simulink model "trackVehicleNewVer7_SonarPath"  (R2017b)
settings: Solver=ode45  StartTime=0.0  StopTime=200  FixedStep=0.1  RelTol=1e-3  EnableMultiTasking=on
PreLoadFcn:
  | RTWConfigurationCB('preloadfcn', bdroot);
InitFcn:
  | parameterVehicle
  | parameterObstacles
  | parameterGNC
  | parameterOccupancyGrid
  | parameterPathPlanner
  | parameterWaypointGenerator
  | miscParameters
StopFcn:
  | myAnimationSonarPath(xActEst,yActEst,thetaActEst,X_array, Y_array, rp1,rp2,sonarInfo, obstaclesArray, OccGrid, gridorig, cellsize)
values from neighbouring files (symbols this model uses):
  b = (92/70)*.31    (= 0.407428571429)    [parameterVehicle.m]
  bDR = b    [parameterGNC.m]
  dcArray = [-100 -11 -10 0 10 11 100]    [parameterVehicle.m]
  dcArrayDR = [-100 -11 -10 0 10 11 100]    [parameterGNC.m]
  eTick = 237    [parameterVehicle.m]
  eTickDR = eTick    [parameterGNC.m]
  KP1 = 10    [parameterGNC.m]
  KP2 = 3    [parameterGNC.m]
  maxgoaldist = 0.2    [parameterWaypointGenerator.m]
  maxwaydist = 0.5    [parameterWaypointGenerator.m]
  obstaclesArray = [0; 0; 0]    [miscParameters.m]
  rl = 0.99*rNominal    (= 0.05242941)    [parameterVehicle.m]
  rNominalDR = rNominal    [parameterGNC.m]
  rp1 = 0.3    [parameterGNC.m]
  rr = 1*rNominal    (= 0.052959)    [parameterVehicle.m]
  Tau1 = 0.01    [parameterGNC.m]
  Tau2 = 0.1    [parameterGNC.m]
  TauEncoderDR = 0.1    [parameterGNC.m]
  thetaIC = 0*(pi/180)    (= 0)    [parameterVehicle.m]
  Tsample = 1/10    (= 0.1)    [parameterGNC.m]
  TsampleEncoder = 1/10    (= 0.1)    [parameterVehicle.m]
  TsampleEncoderDR = TsampleEncoder    [parameterGNC.m]
  Vcom = 3*VmaxDR/4    (= 0.361125)    [parameterGNC.m]
  wArray = [-Vmax, -Vmin, 0, 0,   0, Vmin, Vmax]./rNominal    [parameterVehicle.m]
  wArrayDR = [-Vmax, -Vmin, -Vmin/100, 0,   Vmin/100, Vmin, Vmax]./rNominal    [parameterGNC.m]
  xIC = 0    [parameterVehicle.m]
  yIC = 0    [parameterVehicle.m]
undefined symbols (not defined in the file or in its folder): DiscIntNeverNeededParam, sonar, X, Y, Z
libraries: robotlib x17, simulink x10
CloseFcn:
  | rtwprivate ssgencode ModelCloseRequest track_vehicle6_v2
settings Model: Creator=Dogan  LastModifiedBy=huber
settings DataIOCC: LimitDataPoints=on  SaveFormat=Array  SignalLoggingSaveFormat=ModelDataLogs
settings OptimizationCC: ExpressionDepthLimit=2147483647  InitFltsAndDblsToZero=on  LifeSpan=inf
settings DebuggingCC: SaveWithParameterizedLinksMsg=none  UnderspecifiedInitializationDetection=Classic  MergeDetectMultiDrivingBlocksExec=none  SignalResolutionControl=TryResolveAllWithWarning  SolverPrmCheckMsg=warning  MultiTaskDSMMsg=warning  MultiTaskCondExecSysMsg=none  FcnCallInpInsideContextMsg=warning  StateNameClashWarn=warning  SFUnexpectedBacktrackingDiag=warning  SFNoUnconditionalDefaultTransitionDiag=warning  SFExecutionAtInitializationDiag=none
settings HardwareCC: ProdBitPerLong=64  ProdLargestAtomicFloat=None  ProdHWDeviceType=Intel->x86-64  TargetHWDeviceType=32-bit Generic
settings ModelReferenceCC: PropagateSignalLabelsOutOfModel=off
settings SFSimCC: SimParseCustomCode=off
settings RTWCC: Description=Generic Real-Time Target
settings CodeAppCC: GenerateComments=off  SimulinkBlockComments=off
settings GRTTargetCC: TargetLangStandard=C89/C90 (ANSI)  GeneratePreprocessorConditionals=Disable all
settings ConfigComp: CovMetricSettings=dw  CovHtmlReporting=on  CovSaveCumulativeToWorkspaceVar=on  CovSaveSingleToWorkspaceVar=on  CovExternalEMLEnable=off

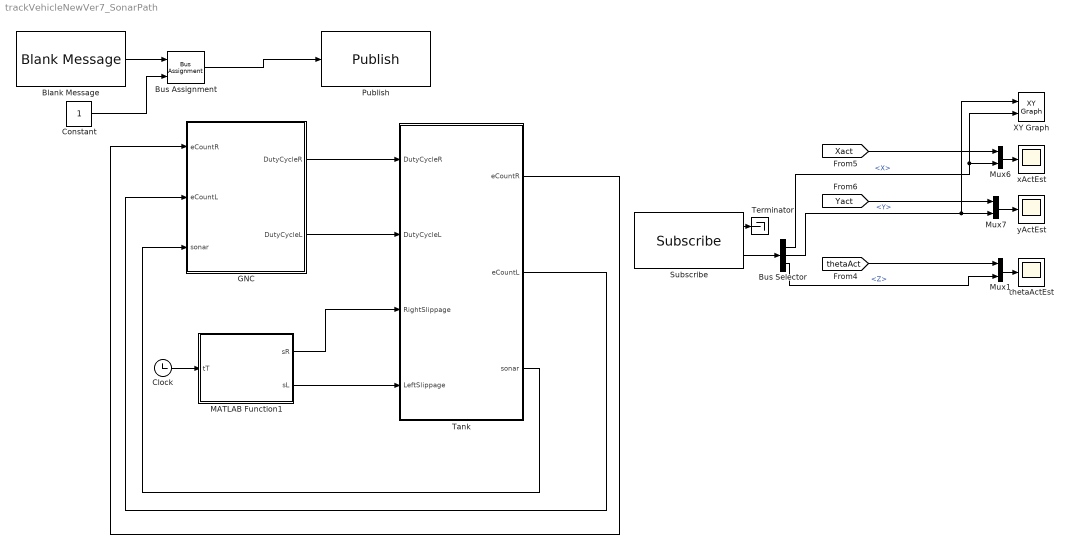
== system trackVehicleNewVer7_SonarPath ==
  Blank Message : robotlib/Blank Message  SourceLibraryInfo=This block requires Robotics System Toolbox  messageType=std_msgs/Bool  SampleTime=-1
      settings: SourceProductBaseCode=RO
  Bus Assignment : BusAssignment  AssignedSignals=Data
  Bus Selector : BusSelector  OutputSignals=X,Y,Z
  Clock : Clock
  Constant : Constant  OutDataTypeStr=boolean
  GNC : Subsystem
  MATLAB Function1 : MATLAB Function  TreatAsAtomicUnit=on
  Mux1 : Mux  Inputs=2
  Mux6 : Mux  Inputs=2
  Mux7 : Mux  Inputs=2
  Publish : robotlib/Publish  SourceLibraryInfo=This block requires Robotics System Toolbox  topicSource=Specify your own  topic=/start  messageType=std_msgs/Bool  messageQueueLength=1
      settings: SourceProductBaseCode=RO
  Subscribe : robotlib/Subscribe  SourceLibraryInfo=This block requires Robotics System Toolbox  topicSource=Specify your own  topic=/odometry  messageType=geometry_msgs/Point  sampleTime=-1  messageQueueLength=1
      settings: SourceProductBaseCode=RO
  Tank : Subsystem
  Terminator : Terminator
  XY Graph : simulink/Sinks/XY Graph  xmin=-1  xmax=9  ymin=-1  ymax=9  st=-1
  thetaActEst : Scope
  xActEst : Scope
  yActEst : Scope
  wires:
  MATLAB Function1/1(sR) -> Tank/3(RightSlippage)
  MATLAB Function1/2(sL) -> Tank/4(LeftSlippage)
  Clock/1 -> MATLAB Function1/1(tT)
  Tank/2(eCountL) -> GNC/2(eCountL)
  Tank/1(eCountR) -> GNC/1(eCountR)
  GNC/1(DutyCycleR) -> Tank/1(DutyCycleR)
  GNC/2(DutyCycleL) -> Tank/2(DutyCycleL)
  Tank/3(sonar) -> GNC/3(sonar)
  Bus Selector/1 -> XY Graph/2, Mux6/2  "<X>"
  Mux6/1 -> xActEst/1
  Bus Selector/2 -> Mux7/2, XY Graph/1  "<Y>"
  [Xact] -> Mux6/1
  [Yact] -> Mux7/1
  Mux7/1 -> yActEst/1
  Bus Selector/3 -> Mux1/2  "<Z>"
  Mux1/1 -> thetaActEst/1
  [thetaAct] -> Mux1/1
  Subscribe/2 -> Bus Selector/1
  Blank Message/1 -> Bus Assignment/1
  Bus Assignment/1 -> Publish/1
  Constant/1 -> Bus Assignment/2
  Subscribe/1 -> Terminator/1

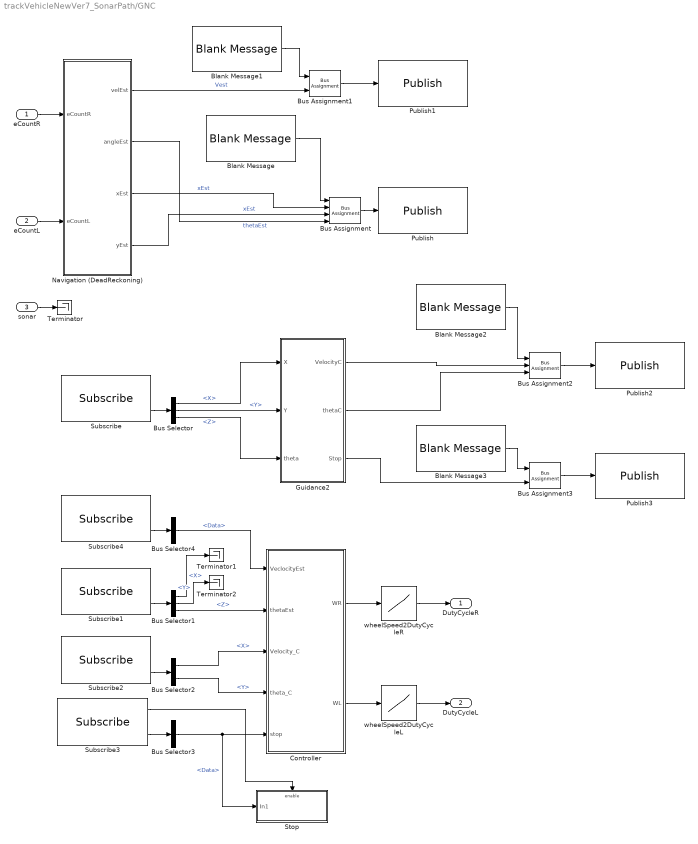
== system trackVehicleNewVer7_SonarPath/GNC ==
  eCountR : Inport
  eCountL : Inport  Port=2
  sonar : Inport  Port=3
  Blank Message : robotlib/Blank Message  SourceLibraryInfo=This block requires Robotics System Toolbox  messageType=geometry_msgs/Point  SampleTime=inf
      settings: SourceProductBaseCode=RO
  Blank Message1 : robotlib/Blank Message  SourceLibraryInfo=This block requires Robotics System Toolbox  messageType=std_msgs/Float64  SampleTime=inf
      settings: SourceProductBaseCode=RO
  Blank Message2 : robotlib/Blank Message  SourceLibraryInfo=This block requires Robotics System Toolbox  messageType=geometry_msgs/Point  SampleTime=inf
      settings: SourceProductBaseCode=RO
  Blank Message3 : robotlib/Blank Message  SourceLibraryInfo=This block requires Robotics System Toolbox  messageType=std_msgs/Bool  SampleTime=inf
      settings: SourceProductBaseCode=RO
  Bus Assignment : BusAssignment  AssignedSignals=X,Y,Z
  Bus Assignment1 : BusAssignment  AssignedSignals=Data
  Bus Assignment2 : BusAssignment  AssignedSignals=X,Y
  Bus Assignment3 : BusAssignment  AssignedSignals=Data
  Bus Selector : BusSelector  OutputSignals=X,Y,Z
  Bus Selector1 : BusSelector  OutputSignals=X,Y,Z
  Bus Selector2 : BusSelector  OutputSignals=X,Y
  Bus Selector3 : BusSelector  OutputSignals=Data
  Bus Selector4 : BusSelector  OutputSignals=Data
  Controller : Subsystem
  Guidance2 : Subsystem
  Navigation (DeadReckoning) : Subsystem
  Publish : robotlib/Publish  SourceLibraryInfo=This block requires Robotics System Toolbox  topicSource=Specify your own  topic=/odometry  messageType=geometry_msgs/Point  messageQueueLength=1
      settings: SourceProductBaseCode=RO
  Publish1 : robotlib/Publish  SourceLibraryInfo=This block requires Robotics System Toolbox  topicSource=Specify your own  topic=/velEst  messageType=std_msgs/Float64  messageQueueLength=1
      settings: SourceProductBaseCode=RO
  Publish2 : robotlib/Publish  SourceLibraryInfo=This block requires Robotics System Toolbox  topicSource=Specify your own  topic=/controlcommands  messageType=geometry_msgs/Point  messageQueueLength=1
      settings: SourceProductBaseCode=RO
  Publish3 : robotlib/Publish  SourceLibraryInfo=This block requires Robotics System Toolbox  topicSource=Specify your own  topic=/stop  messageType=std_msgs/Bool  messageQueueLength=1
      settings: SourceProductBaseCode=RO
  Stop : Subsystem  TreatAsAtomicUnit=on
  Subscribe : robotlib/Subscribe  SourceLibraryInfo=This block requires Robotics System Toolbox  topicSource=Specify your own  topic=/odometry  messageType=geometry_msgs/Point  sampleTime=-1  messageQueueLength=1
      settings: SourceProductBaseCode=RO
  Subscribe1 : robotlib/Subscribe  SourceLibraryInfo=This block requires Robotics System Toolbox  topicSource=Specify your own  topic=/odometry  messageType=geometry_msgs/Point  sampleTime=-1  messageQueueLength=1
      settings: SourceProductBaseCode=RO
  Subscribe2 : robotlib/Subscribe  SourceLibraryInfo=This block requires Robotics System Toolbox  topicSource=Specify your own  topic=/controlcommands  messageType=geometry_msgs/Point  sampleTime=-1  messageQueueLength=1
      settings: SourceProductBaseCode=RO
  Subscribe3 : robotlib/Subscribe  SourceLibraryInfo=This block requires Robotics System Toolbox  topicSource=Specify your own  topic=/stop  messageType=std_msgs/Bool  sampleTime=-1  messageQueueLength=1
      settings: SourceProductBaseCode=RO
  Subscribe4 : robotlib/Subscribe  SourceLibraryInfo=This block requires Robotics System Toolbox  topicSource=Specify your own  topic=/velEst  messageType=std_msgs/Float64  sampleTime=-1  messageQueueLength=1
      settings: SourceProductBaseCode=RO
  Terminator : Terminator
  Terminator1 : Terminator
  Terminator2 : Terminator
  wheelSpeed2DutyCycleL : Lookup  InputValues=wArrayDR  Table=dcArrayDR  LookUpMeth=Interpolation-Use End Values
  wheelSpeed2DutyCycleR : Lookup  InputValues=wArrayDR  Table=dcArrayDR  LookUpMeth=Interpolation-Use End Values
  DutyCycleR : Outport
  DutyCycleL : Outport  Port=2
  wires:
  wheelSpeed2DutyCycleL/1 -> DutyCycleL/1
  Controller/2(WL) -> wheelSpeed2DutyCycleL/1
  wheelSpeed2DutyCycleR/1 -> DutyCycleR/1
  Guidance2/2(thetaC) -> Bus Assignment2/3
  Guidance2/1(VelocityC) -> Bus Assignment2/2
  eCountR/1 -> Navigation (DeadReckoning)/1(eCountR)
  eCountL/1 -> Navigation (DeadReckoning)/2(eCountL)
  Navigation (DeadReckoning)/1(velEst) -> Bus Assignment1/2  "Vest"
  Navigation (DeadReckoning)/2(angleEst) -> Bus Assignment/4  "thetaEst"
  Navigation (DeadReckoning)/3(xEst) -> Bus Assignment/2  "xEst"
  Navigation (DeadReckoning)/4(yEst) -> Bus Assignment/3  "xEst"
  Controller/1(WR) -> wheelSpeed2DutyCycleR/1
  Guidance2/3(Stop) -> Bus Assignment3/2
  sonar/1 -> Terminator/1
  Bus Assignment/1 -> Publish/1
  Blank Message/1 -> Bus Assignment/1
  Blank Message1/1 -> Bus Assignment1/1
  Bus Assignment1/1 -> Publish1/1
  Subscribe/2 -> Bus Selector/1
  Bus Selector/1 -> Guidance2/1(X)  "<X>"
  Bus Selector/2 -> Guidance2/2(Y)  "<Y>"
  Bus Selector/3 -> Guidance2/3(theta)  "<Z>"
  Bus Assignment2/1 -> Publish2/1
  Blank Message2/1 -> Bus Assignment2/1
  Subscribe1/2 -> Bus Selector1/1
  Bus Selector1/3 -> Controller/2(thetaEst)  "<Z>"
  Bus Selector1/1 -> Terminator1/1  "<X>"
  Bus Selector1/2 -> Terminator2/1  "<Y>"
  Subscribe2/2 -> Bus Selector2/1
  Bus Selector2/1 -> Controller/3(Velocity_C)  "<X>"
  Bus Selector2/2 -> Controller/4(theta_C)  "<Y>"
  Bus Assignment3/1 -> Publish3/1
  Blank Message3/1 -> Bus Assignment3/1
  Subscribe3/2 -> Bus Selector3/1
  Bus Selector3/1 -> Stop/1(In1), Controller/5(stop)  "<Data>"
  Subscribe4/2 -> Bus Selector4/1
  Bus Selector4/1 -> Controller/1(VeclocityEst)  "<Data>"
  Subscribe3/1 -> Stop/Enable

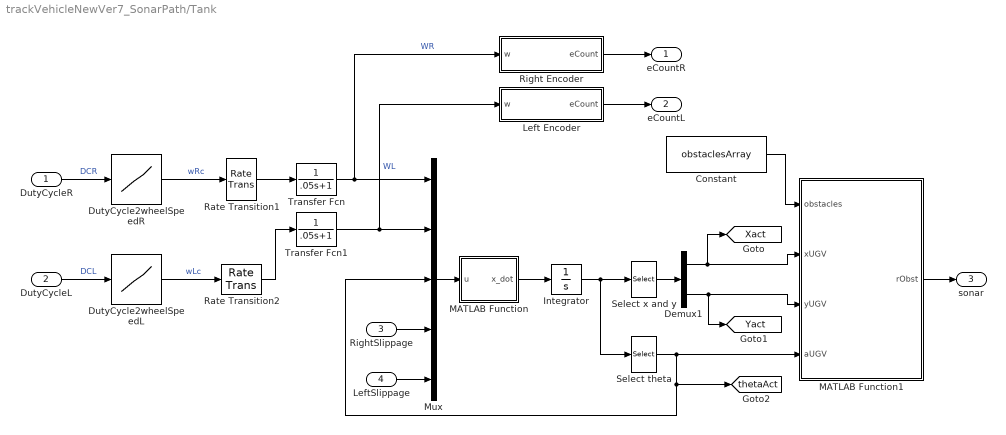
== system trackVehicleNewVer7_SonarPath/Tank ==
  DutyCycleR : Inport
  DutyCycleL : Inport  Port=2
  RightSlippage : Inport  Port=3
  LeftSlippage : Inport  Port=4
  Constant : Constant  Value=obstaclesArray
  Demux1 : Demux  Outputs=2
  DutyCycle2wheelSpeedL : Lookup  InputValues=dcArray  Table=wArray  LookUpMeth=Interpolation-Use End Values
  DutyCycle2wheelSpeedR : Lookup  InputValues=dcArray  Table=wArray  LookUpMeth=Interpolation-Use End Values
  Integrator : Integrator  InitialCondition=[xIC; yIC ; thetaIC]
  Left Encoder : Subsystem
  MATLAB Function : MATLAB Function  TreatAsAtomicUnit=on
  MATLAB Function1 : MATLAB Function  TreatAsAtomicUnit=on  SystemSampleTime=sonar.Ts
  Mux : Mux  Inputs=5
  Rate Transition1 : RateTransition
  Rate Transition2 : RateTransition
  Right Encoder : Subsystem
  Select theta : Selector  InputPortWidth=3  IndexOptions=Index vector (dialog)  Indices=3  OutputSizes=1
  Select x and y : Selector  InputPortWidth=3  IndexOptions=Index vector (dialog)  Indices=[1 2]  OutputSizes=1
  Transfer Fcn : TransferFcn  Denominator=[.05 1]
  Transfer Fcn1 : TransferFcn  Denominator=[.05 1]
  eCountR : Outport
  eCountL : Outport  Port=2
  sonar : Outport  Port=3
  tag scope: Xact=global, Yact=global, thetaAct=global
  wires:
  DutyCycleL/1 -> DutyCycle2wheelSpeedL/1  "DCL"
  DutyCycleR/1 -> DutyCycle2wheelSpeedR/1  "DCR"
  DutyCycle2wheelSpeedL/1 -> Rate Transition2/1  "wLc"
  DutyCycle2wheelSpeedR/1 -> Rate Transition1/1  "wRc"
  Left Encoder/1(eCount) -> eCountL/1
  Right Encoder/1(eCount) -> eCountR/1
  Rate Transition2/1 -> Transfer Fcn1/1
  Rate Transition1/1 -> Transfer Fcn/1
  Demux1/2 -> [Yact], MATLAB Function1/3(yUGV)
  Demux1/1 -> [Xact], MATLAB Function1/2(xUGV)
  Select x and y/1 -> Demux1/1
  MATLAB Function/1(x_dot) -> Integrator/1
  Select theta/1 -> [thetaAct], Mux/3, MATLAB Function1/4(aUGV)
  Transfer Fcn1/1 -> Left Encoder/1(w), Mux/2  "WL"
  Transfer Fcn/1 -> Right Encoder/1(w), Mux/1  "WR"
  LeftSlippage/1 -> Mux/5
  RightSlippage/1 -> Mux/4
  Mux/1 -> MATLAB Function/1(u)
  Integrator/1 -> Select theta/1, Select x and y/1
  Constant/1 -> MATLAB Function1/1(obstacles)
  MATLAB Function1/1(rObst) -> sonar/1

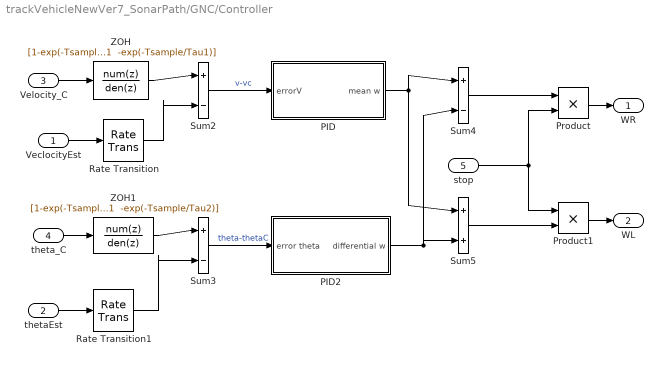
== system trackVehicleNewVer7_SonarPath/GNC/Controller ==
  VeclocityEst : Inport
  thetaEst : Inport  Port=2
  Velocity_C : Inport  Port=3
  theta_C : Inport  Port=4
  stop : Inport  Port=5
  PID : Subsystem
  PID2 : Subsystem
  Product : Product  RndMeth=Zero
  Product1 : Product  RndMeth=Zero
  Rate Transition : RateTransition  Deterministic=off
  Rate Transition1 : RateTransition  Deterministic=off
  Sum2 : Sum  Inputs=|+|-|  SampleTime=Tsample
  Sum3 : Sum  Inputs=|+|-|  SampleTime=Tsample
  Sum4 : Sum  Inputs=+|-
  Sum5 : Sum  Inputs=+|+
  ZOH : DiscreteTransferFcn  Numerator=[1-exp(-Tsample/Tau1)]  Denominator="[1  -exp(-Tsample/Tau1)]"  SampleTime=Tsample
  ZOH1 : DiscreteTransferFcn  Numerator=[1-exp(-Tsample/Tau2)]  Denominator="[1  -exp(-Tsample/Tau2)]"  SampleTime=Tsample
  WR : Outport
  WL : Outport  Port=2
  wires:
  Rate Transition1/1 -> Sum3/2
  ZOH1/1 -> Sum3/1
  Rate Transition/1 -> Sum2/2
  ZOH/1 -> Sum2/1
  Sum3/1 -> PID2/1(error theta)  "theta-thetaC"
  Sum2/1 -> PID/1(errorV)  "v-vc"
  VeclocityEst/1 -> Rate Transition/1
  Velocity_C/1 -> ZOH/1
  thetaEst/1 -> Rate Transition1/1
  theta_C/1 -> ZOH1/1
  PID/1(mean w) -> Sum4/1, Sum5/1
  PID2/1(differential w) -> Sum4/2, Sum5/2
  Sum4/1 -> Product/1
  stop/1 -> Product1/1, Product/2
  Sum5/1 -> Product1/2
  Product/1 -> WR/1
  Product1/1 -> WL/1

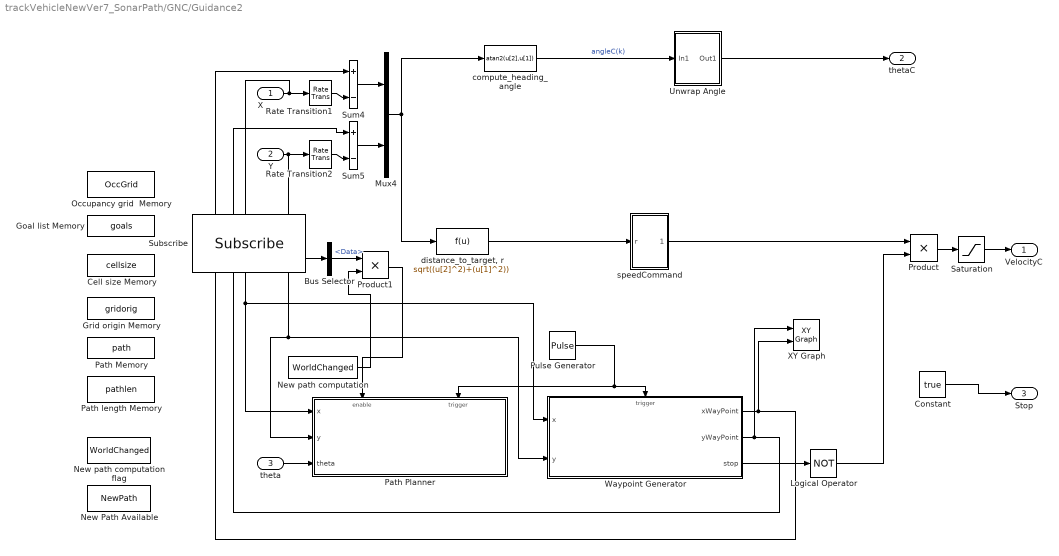
== system trackVehicleNewVer7_SonarPath/GNC/Guidance2 ==
  X : Inport
  Y : Inport  Port=2
  theta : Inport  Port=3
  Bus Selector : BusSelector  OutputSignals=Data
  Cell size Memory : DataStoreMemory  DataStoreName=cellsize  ReadBeforeWriteMsg=warning  WriteAfterWriteMsg=warning  WriteAfterReadMsg=warning  InitialValue=cellsize  VectorParams1D=off  ShowAdditionalParam=off
  Constant : Constant  Value=true
  Goal list Memory : DataStoreMemory  DataStoreName=goals  ReadBeforeWriteMsg=warning  WriteAfterWriteMsg=warning  WriteAfterReadMsg=warning  InitialValue=goals  VectorParams1D=off  ShowAdditionalParam=off
  Grid origin Memory : DataStoreMemory  DataStoreName=gridorig  InitialValue=gridorig  VectorParams1D=off  ShowAdditionalParam=off
  Logical Operator : Logic  Operator=NOT  AllPortsSameDT=off
  Mux4 : Mux  Inputs=2
  New Path Available : DataStoreMemory  DataStoreName=NewPath  ReadBeforeWriteMsg=warning  WriteAfterWriteMsg=warning  WriteAfterReadMsg=warning  VectorParams1D=off  ShowAdditionalParam=off
  New path computation : DataStoreRead  DataStoreName=WorldChanged
  New path computation flag : DataStoreMemory  DataStoreName=WorldChanged  InitialValue=WorldChanged  VectorParams1D=off  ShowAdditionalParam=off
  Occupancy grid  Memory : DataStoreMemory  DataStoreName=OccGrid  InitialValue=OccGrid  VectorParams1D=off  ShowAdditionalParam=off
  Path Memory : DataStoreMemory  DataStoreName=path  InitialValue=path  VectorParams1D=off  ShowAdditionalParam=off
  Path Planner : Subsystem
  Path length Memory : DataStoreMemory  DataStoreName=pathlen  InitialValue=pathlen  VectorParams1D=off  ShowAdditionalParam=off
  Product : Product  RndMeth=Zero
  Product1 : Product
  Pulse Generator : DiscretePulseGenerator  PulseType=Time based  Period=0.1  PulseWidth=5
  Rate Transition1 : RateTransition
  Rate Transition2 : RateTransition
  Saturation : Saturate  UpperLimit=Vcom  LowerLimit=0  SampleTime=Tsample
  Subscribe : robotlib/Subscribe  SourceLibraryInfo=This block requires Robotics System Toolbox  topicSource=Specify your own  topic=/start  messageType=std_msgs/Bool  sampleTime=-1  messageQueueLength=1
      settings: SourceProductBaseCode=RO
  Sum4 : Sum  Inputs=|+|-|
  Sum5 : Sum  Inputs=|+|-|
  Unwrap Angle : Subsystem
  Waypoint Generator : Subsystem
  XY Graph : simulink/Sinks/XY Graph  xmin=-1  xmax=9  ymin=-1  ymax=9  st=-1
  compute_heading_angle : Fcn  Expr=atan2(u[2],u[1])  SampleTime=Tsample
  "distance_to_target, r" : Fcn  Expr=sqrt((u[2]^2)+(u[1]^2))  SampleTime=Tsample
  speedCommand : Subsystem
  VelocityC : Outport
  thetaC : Outport  Port=2
  Stop : Outport  Port=3
  wires:
  Product/1 -> Saturation/1
  Rate Transition2/1 -> Sum5/2
  Rate Transition1/1 -> Sum4/2
  Unwrap Angle/1(Out1) -> thetaC/1
  Saturation/1 -> VelocityC/1
  Sum5/1 -> Mux4/2
  Y/1 -> Rate Transition2/1, Path Planner/2(y), Waypoint Generator/2(y)
  X/1 -> Rate Transition1/1, Waypoint Generator/1(x), Path Planner/1(x)
  Mux4/1 -> "distance_to_target, r"/1, compute_heading_angle/1
  "distance_to_target, r"/1 -> speedCommand/1(r)
  Sum4/1 -> Mux4/1
  compute_heading_angle/1 -> Unwrap Angle/1(In1)  "angleC(k)"
  speedCommand/1(Vdes) -> Product/1
  theta/1 -> Path Planner/3(theta)
  New path computation/1 -> Product1/2
  Waypoint Generator/1(xWayPoint) -> XY Graph/2, Sum4/1
  Waypoint Generator/2(yWayPoint) -> XY Graph/1, Sum5/1
  Waypoint Generator/3(stop) -> Logical Operator/1
  Logical Operator/1 -> Product/2
  Pulse Generator/1 -> Path Planner/Trigger, Waypoint Generator/Trigger
  Constant/1 -> Stop/1
  Product1/1 -> Path Planner/Enable
  Subscribe/2 -> Bus Selector/1
  Bus Selector/1 -> Product1/1  "<Data>"

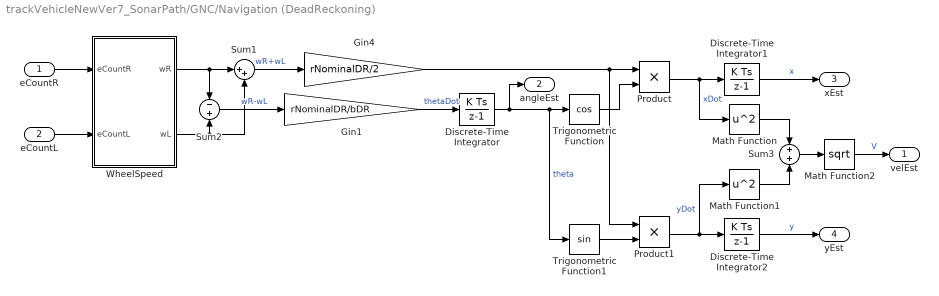
== system trackVehicleNewVer7_SonarPath/GNC/Navigation (DeadReckoning) ==
  eCountR : Inport
  eCountL : Inport  Port=2
  Discrete-Time Integrator : DiscreteIntegrator  SampleTime=TsampleEncoderDR  ICPrevOutput=DiscIntNeverNeededParam  ICPrevScaledInput=DiscIntNeverNeededParam
  Discrete-Time Integrator1 : DiscreteIntegrator  SampleTime=TsampleEncoderDR  ICPrevOutput=DiscIntNeverNeededParam  ICPrevScaledInput=DiscIntNeverNeededParam
  Discrete-Time Integrator2 : DiscreteIntegrator  SampleTime=TsampleEncoderDR  ICPrevOutput=DiscIntNeverNeededParam  ICPrevScaledInput=DiscIntNeverNeededParam
  Gin1 : Gain  Gain=rNominalDR/bDR  OutDataTypeStr=double
  Gin4 : Gain  Gain=rNominalDR/2  OutDataTypeStr=double
  Math Function : Math  Operator=square  SaturateOnIntegerOverflow=on
  Math Function1 : Math  Operator=square  SaturateOnIntegerOverflow=on
  Math Function2 : Math  Operator=sqrt  OutputSignalType=real  SaturateOnIntegerOverflow=on
  Product : Product  RndMeth=Zero
  Product1 : Product  RndMeth=Zero
  Sum1 : Sum  Inputs=|++
  Sum2 : Sum  Inputs=-|+
  Sum3 : Sum  Inputs=+|+
  Trigonometric Function : Trigonometry  Operator=cos  OutputSignalType=real
  Trigonometric Function1 : Trigonometry  OutputSignalType=real
  WheelSpeed : Subsystem
  velEst : Outport
  angleEst : Outport  Port=2
  xEst : Outport  Port=3
  yEst : Outport  Port=4
  wires:
  eCountR/1 -> WheelSpeed/1(eCountR)
  eCountL/1 -> WheelSpeed/2(eCountL)
  WheelSpeed/2(wL) -> Sum1/2, Sum2/2
  WheelSpeed/1(wR) -> Sum1/1, Sum2/1
  Sum1/1 -> Gin4/1  "wR+wL"
  Sum2/1 -> Gin1/1  "wR-wL"
  Gin1/1 -> Discrete-Time Integrator/1  "thetaDot"
  Discrete-Time Integrator/1 -> Trigonometric Function/1, Trigonometric Function1/1, angleEst/1  "theta"
  Trigonometric Function/1 -> Product/2
  Gin4/1 -> Product/1, Product1/1
  Trigonometric Function1/1 -> Product1/2
  Product/1 -> Discrete-Time Integrator1/1, Math Function/1  "xDot"
  Product1/1 -> Discrete-Time Integrator2/1, Math Function1/1  "yDot"
  Discrete-Time Integrator1/1 -> xEst/1  "x"
  Discrete-Time Integrator2/1 -> yEst/1  "y"
  Math Function/1 -> Sum3/1
  Math Function1/1 -> Sum3/2
  Sum3/1 -> Math Function2/1
  Math Function2/1 -> velEst/1  "V"

== system trackVehicleNewVer7_SonarPath/GNC/Stop ==
  In1 : Inport
  Enable : EnablePort
  Compare To Zero : simulink/Logic and Bit Operations/Compare To Zero  relop===  OutDataTypeStr=boolean
  Stop Simulation : Stop
  wires:
  Compare To Zero/1 -> Stop Simulation/1
  In1/1 -> Compare To Zero/1

== system trackVehicleNewVer7_SonarPath/Tank/Left Encoder ==
  w : Inport
  Rate Transition1 : RateTransition
  WheelAngleL : Integrator
  angle2tick2 : Gain  Gain=eTick*rl  OutDataTypeStr=int16  SampleTime=TsampleEncoder
  eCount : Outport
  wires:
  Rate Transition1/1 -> angle2tick2/1
  angle2tick2/1 -> eCount/1  "eCountL"
  w/1 -> WheelAngleL/1
  WheelAngleL/1 -> Rate Transition1/1  "gammaL"

== system trackVehicleNewVer7_SonarPath/Tank/Right Encoder ==
  w : Inport
  Rate Transition1 : RateTransition
  WheelAngleR : Integrator
  angle2tick1 : Gain  Gain=eTick*rr  OutDataTypeStr=int16  SampleTime=TsampleEncoder
  eCount : Outport
  wires:
  Rate Transition1/1 -> angle2tick1/1
  angle2tick1/1 -> eCount/1  "eCountR"
  w/1 -> WheelAngleR/1
  WheelAngleR/1 -> Rate Transition1/1  "gammaR"

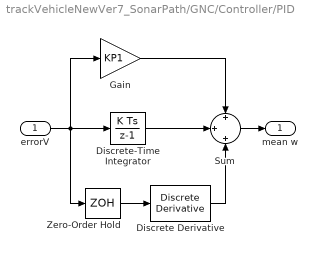
== system trackVehicleNewVer7_SonarPath/GNC/Controller/PID ==
  errorV : Inport
  Discrete Derivative : simulink/Discrete/Discrete Derivative  gainval=KD1  ICPrevScaledInput=0.0  InputProcessing=Inherited  OutMin=[]  OutMax=[]  OutDataType=sfix(16)  OutScaling=2^-10  DoSatur=off
  Discrete-Time Integrator : DiscreteIntegrator  gainval=KI1  SampleTime=Tsample  ICPrevOutput=DiscIntNeverNeededParam  ICPrevScaledInput=DiscIntNeverNeededParam
  Gain : Gain  Gain=KP1  SampleTime=Tsample
  Sum : Sum  Inputs=+|+|+
  Zero-Order Hold : ZeroOrderHold  SampleTime=Tsample
  mean w : Outport
  wires:
  Sum/1 -> mean w/1
  errorV/1 -> Zero-Order Hold/1, Gain/1, Discrete-Time Integrator/1
  Gain/1 -> Sum/1
  Discrete-Time Integrator/1 -> Sum/2
  Zero-Order Hold/1 -> Discrete Derivative/1
  Discrete Derivative/1 -> Sum/3

== system trackVehicleNewVer7_SonarPath/GNC/Controller/PID2 ==
  error theta : Inport
  Discrete Derivative1 : simulink/Discrete/Discrete Derivative  gainval=KD2  ICPrevScaledInput=0.0  InputProcessing=Inherited  OutMin=[]  OutMax=[]  OutDataType=sfix(16)  OutScaling=2^-10  DoSatur=off
  Discrete-Time Integrator1 : DiscreteIntegrator  gainval=KI2  SampleTime=Tsample  ICPrevOutput=DiscIntNeverNeededParam  ICPrevScaledInput=DiscIntNeverNeededParam
  Gain1 : Gain  Gain=KP2  SampleTime=Tsample
  Sum1 : Sum  Inputs=+|+|+
  Zero-Order Hold1 : ZeroOrderHold  SampleTime=Tsample
  differential w : Outport
  wires:
  Sum1/1 -> differential w/1
  Gain1/1 -> Sum1/1
  Discrete-Time Integrator1/1 -> Sum1/2
  error theta/1 -> Zero-Order Hold1/1, Discrete-Time Integrator1/1, Gain1/1
  Zero-Order Hold1/1 -> Discrete Derivative1/1
  Discrete Derivative1/1 -> Sum1/3

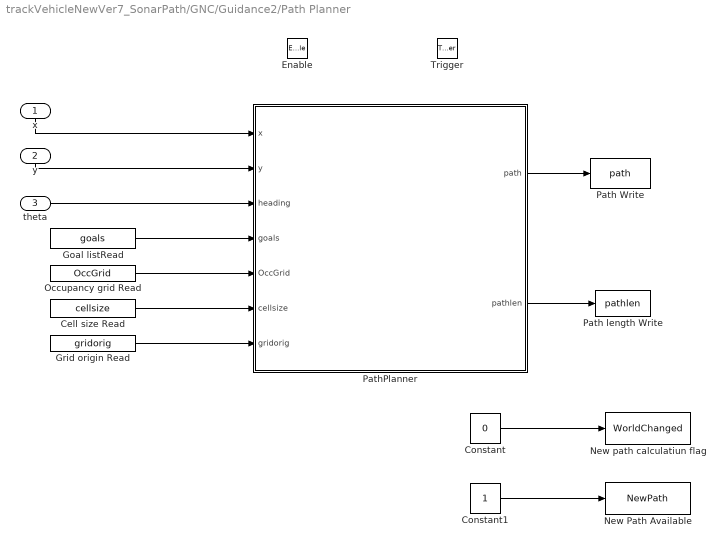
== system trackVehicleNewVer7_SonarPath/GNC/Guidance2/Path Planner ==
  x : Inport
  y : Inport  Port=2
  theta : Inport  Port=3
  Enable : EnablePort  ZeroCross=off
  Trigger : TriggerPort  VariantControl=(inherit)  PortDimensions=1
  Cell size Read : DataStoreRead  DataStoreName=cellsize
  Constant : Constant  Value=0  VectorParams1D=off
  Constant1 : Constant
  Goal listRead : DataStoreRead  DataStoreName=goals
  Grid origin Read : DataStoreRead  DataStoreName=gridorig
  New Path Available : DataStoreWrite  DataStoreName=NewPath
  New path calculatiun flag : DataStoreWrite  DataStoreName=WorldChanged  DataStoreElements=WorldChanged
  Occupancy grid Read : DataStoreRead  DataStoreName=OccGrid
  Path Write : DataStoreWrite  DataStoreName=path
  Path length Write : DataStoreWrite  DataStoreName=pathlen
  PathPlanner : MATLAB Function  TreatAsAtomicUnit=on
  wires:
  theta/1 -> PathPlanner/3(heading)
  Grid origin Read/1 -> PathPlanner/7(gridorig)
  Cell size Read/1 -> PathPlanner/6(cellsize)
  Occupancy grid Read/1 -> PathPlanner/5(OccGrid)
  Goal listRead/1 -> PathPlanner/4(goals)
  x/1 -> PathPlanner/1(x)
  PathPlanner/1(path) -> Path Write/1
  Constant/1 -> New path calculatiun flag/1
  PathPlanner/2(pathlen) -> Path length Write/1
  Constant1/1 -> New Path Available/1
  y/1 -> PathPlanner/2(y)

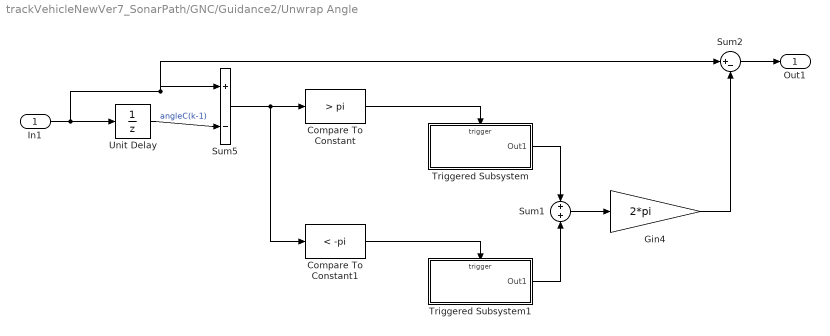
== system trackVehicleNewVer7_SonarPath/GNC/Guidance2/Unwrap Angle ==
  In1 : Inport
  Compare To Constant : simulink/Logic and Bit Operations/Compare To Constant  relop=>  const=pi  OutDataTypeStr=uint8  ZeroCross=off
  Compare To Constant1 : simulink/Logic and Bit Operations/Compare To Constant  relop=<  const=-pi  OutDataTypeStr=uint8  ZeroCross=off
  Gin4 : Gain  Gain=2*pi  OutDataTypeStr=double  SampleTime=Tsample
  Sum1 : Sum  Inputs=+|+
  Sum2 : Sum  Inputs=|+-
  Sum5 : Sum  Inputs=|+|-|
  Triggered Subsystem : Subsystem  TreatAsAtomicUnit=on
  Triggered Subsystem1 : Subsystem  TreatAsAtomicUnit=on
  Unit Delay : UnitDelay  SampleTime=Tsample
  Out1 : Outport
  wires:
  Gin4/1 -> Sum2/2
  Sum2/1 -> Out1/1
  Sum1/1 -> Gin4/1
  Triggered Subsystem1/1(Out1) -> Sum1/2
  Triggered Subsystem/1(Out1) -> Sum1/1
  Compare To Constant/1 -> Triggered Subsystem/Trigger
  Compare To Constant1/1 -> Triggered Subsystem1/Trigger
  Sum5/1 -> Compare To Constant1/1, Compare To Constant/1
  Unit Delay/1 -> Sum5/2  "angleC(k-1)"
  In1/1 -> Sum2/1, Sum5/1, Unit Delay/1

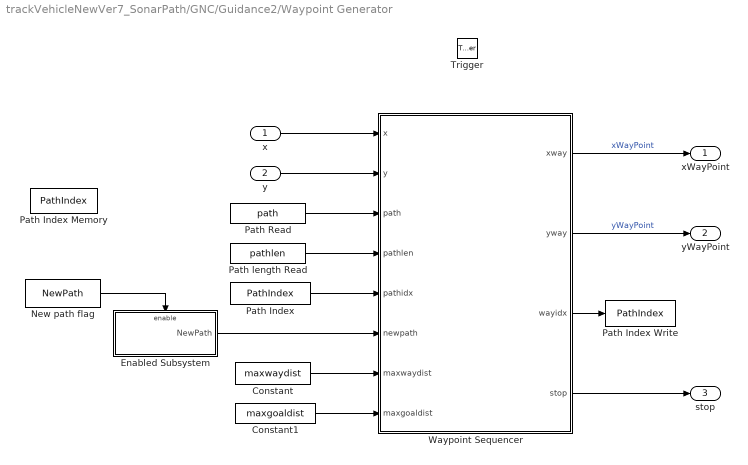
== system trackVehicleNewVer7_SonarPath/GNC/Guidance2/Waypoint Generator ==
  x : Inport
  y : Inport  Port=2
  Trigger : TriggerPort  VariantControl=(inherit)  PortDimensions=1
  Constant : Constant  Value=maxwaydist  VectorParams1D=off
  Constant1 : Constant  Value=maxgoaldist
  Enabled Subsystem : Subsystem  TreatAsAtomicUnit=on
  New path flag : DataStoreRead  DataStoreName=NewPath
  Path Index : DataStoreRead  DataStoreName=PathIndex
  Path Index Memory : DataStoreMemory  DataStoreName=PathIndex  InitialValue=1  VectorParams1D=off  ShowAdditionalParam=off
  Path Index Write : DataStoreWrite  DataStoreName=PathIndex
  Path Read : DataStoreRead  DataStoreName=path
  Path length Read : DataStoreRead  DataStoreName=pathlen
  Waypoint Sequencer : MATLAB Function  TreatAsAtomicUnit=on
  xWayPoint : Outport
  yWayPoint : Outport  Port=2
  stop : Outport  Port=3
  wires:
  Waypoint Sequencer/2(yway) -> yWayPoint/1  "yWayPoint"
  Waypoint Sequencer/1(xway) -> xWayPoint/1  "xWayPoint"
  Path Read/1 -> Waypoint Sequencer/3(path)
  Path length Read/1 -> Waypoint Sequencer/4(pathlen)
  Path Index/1 -> Waypoint Sequencer/5(pathidx)
  Waypoint Sequencer/3(wayidx) -> Path Index Write/1
  New path flag/1 -> Enabled Subsystem/Enable
  Enabled Subsystem/1(NewPath) -> Waypoint Sequencer/6(newpath)
  Waypoint Sequencer/4(stop) -> stop/1
  Constant/1 -> Waypoint Sequencer/7(maxwaydist)
  Constant1/1 -> Waypoint Sequencer/8(maxgoaldist)
  y/1 -> Waypoint Sequencer/2(y)
  x/1 -> Waypoint Sequencer/1(x)

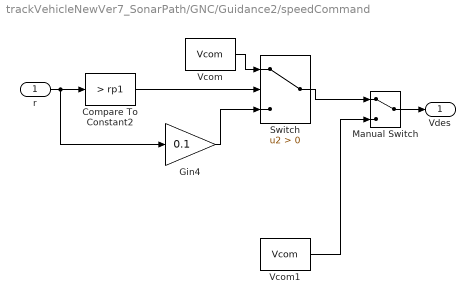
== system trackVehicleNewVer7_SonarPath/GNC/Guidance2/speedCommand ==
  r : Inport
  Compare To Constant2 : simulink/Logic and Bit Operations/Compare To Constant  relop=>  const=rp1  OutDataTypeStr=uint8  ZeroCross=off
  Gin4 : Gain  Gain=0.1  SampleTime=Tsample
  Manual Switch : ManualSwitch
  Switch : Switch  Criteria=u2 > Threshold
  Vcom : Constant  Value=Vcom  SampleTime=Tsample
  Vcom1 : Constant  Value=Vcom  SampleTime=Tsample
  Vdes : Outport
  wires:
  Manual Switch/1 -> Vdes/1
  r/1 -> Gin4/1, Compare To Constant2/1
  Gin4/1 -> Switch/3
  Switch/1 -> Manual Switch/1
  Vcom1/1 -> Manual Switch/2
  Vcom/1 -> Switch/1
  Compare To Constant2/1 -> Switch/2

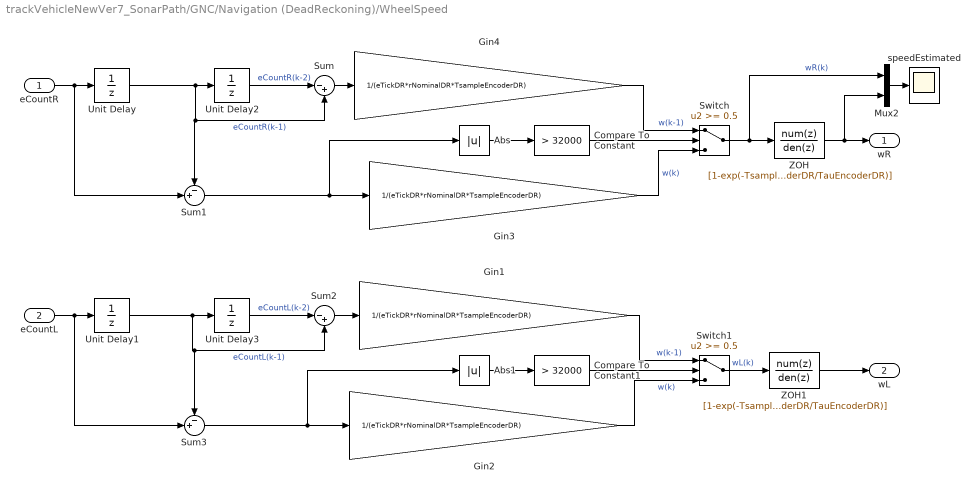
== system trackVehicleNewVer7_SonarPath/GNC/Navigation (DeadReckoning)/WheelSpeed ==
  eCountR : Inport
  eCountL : Inport  Port=2
  Abs : Abs
  Abs1 : Abs
  Compare To Constant : simulink/Logic and Bit Operations/Compare To Constant  relop=>  const=32000  OutDataTypeStr=uint8  ZeroCross=off
  Compare To Constant1 : simulink/Logic and Bit Operations/Compare To Constant  relop=>  const=32000  OutDataTypeStr=uint8  ZeroCross=off
  Gin{1..4} (4 alike) : Gain  Gain=1/(eTickDR*rNominalDR*TsampleEncoderDR)  OutDataTypeStr=double  SampleTime=TsampleEncoderDR
  Mux2 : Mux  Inputs=2
  Sum : Sum  Inputs=|-+
  Sum1 : Sum  Inputs=-+|
  Sum2 : Sum  Inputs=|-+
  Sum3 : Sum  Inputs=-+|
  Switch : Switch  Threshold=0.5
  Switch1 : Switch  Threshold=0.5
  Unit Delay{,1..3} (4 alike) : UnitDelay  SampleTime=TsampleEncoderDR
  ZOH : DiscreteTransferFcn  Numerator=[1-exp(-TsampleEncoderDR/TauEncoderDR)]  Denominator="[1  -exp(-TsampleEncoderDR/TauEncoderDR)]"  SampleTime=TsampleEncoderDR
  ZOH1 : DiscreteTransferFcn  Numerator=[1-exp(-TsampleEncoderDR/TauEncoderDR)]  Denominator="[1  -exp(-TsampleEncoderDR/TauEncoderDR)]"  SampleTime=TsampleEncoderDR
  speedEstimated : Scope
  wR : Outport
  wL : Outport  Port=2
  wires:
  eCountR/1 -> Unit Delay/1, Sum1/2
  Unit Delay/1 -> Unit Delay2/1, Sum/2, Sum1/1  "eCountR(k-1)"
  Unit Delay2/1 -> Sum/1  "eCountR(k-2)"
  Sum/1 -> Gin4/1
  Sum1/1 -> Abs/1, Gin3/1
  Gin4/1 -> Switch/1  "w(k-1)"
  Gin3/1 -> Switch/3  "w(k)"
  Abs/1 -> Compare To Constant/1
  Compare To Constant/1 -> Switch/2
  eCountL/1 -> Sum3/2, Unit Delay1/1
  Unit Delay1/1 -> Sum3/1, Sum2/2, Unit Delay3/1  "eCountL(k-1)"
  Unit Delay3/1 -> Sum2/1  "eCountL(k-2)"
  Sum2/1 -> Gin1/1
  Sum3/1 -> Abs1/1, Gin2/1
  Gin1/1 -> Switch1/1  "w(k-1)"
  Gin2/1 -> Switch1/3  "w(k)"
  Abs1/1 -> Compare To Constant1/1
  Compare To Constant1/1 -> Switch1/2
  Switch/1 -> ZOH/1, Mux2/1  "wR(k)"
  Switch1/1 -> ZOH1/1  "wL(k)"
  ZOH/1 -> wR/1, Mux2/2
  ZOH1/1 -> wL/1
  Mux2/1 -> speedEstimated/1

== system trackVehicleNewVer7_SonarPath/GNC/Guidance2/Unwrap Angle/Triggered Subsystem ==
  Trigger : TriggerPort  VariantControl=(inherit)
  Sum3 : Sum  OutDataTypeStr=int32
  Unit Delay : UnitDelay  SampleTime=-1
  countIncrement : Constant  OutDataTypeStr=int32  SampleTime=-1
  Out1 : Outport  OutDataTypeStr=int32  InitialOutput=0
  wires:
  Sum3/1 -> Unit Delay/1, Out1/1
  Unit Delay/1 -> Sum3/1
  countIncrement/1 -> Sum3/2

== system trackVehicleNewVer7_SonarPath/GNC/Guidance2/Unwrap Angle/Triggered Subsystem1 ==
  Trigger : TriggerPort  VariantControl=(inherit)
  Sum3 : Sum  Inputs=+-  OutDataTypeStr=int32
  Unit Delay : UnitDelay  SampleTime=-1
  countIncrement : Constant  OutDataTypeStr=int32  SampleTime=-1
  Out1 : Outport  OutDataTypeStr=int32  InitialOutput=0
  wires:
  countIncrement/1 -> Sum3/2
  Unit Delay/1 -> Sum3/1
  Sum3/1 -> Unit Delay/1, Out1/1

== system trackVehicleNewVer7_SonarPath/GNC/Guidance2/Waypoint Generator/Enabled Subsystem ==
  Enable : EnablePort  ZeroCross=off
  Constant : Constant
  Constant1 : Constant  Value=0
  New path flag : DataStoreWrite  DataStoreName=NewPath
  NewPath : Outport  OutputWhenDisabled=reset  InitialOutput=0
  wires:
  Constant/1 -> NewPath/1
  Constant1/1 -> New path flag/1

== matlab function trackVehicleNewVer7_SonarPath/Tank/MATLAB Function ==
  data: u input; x_dot output; b parameter; rr parameter; rl parameter
function x_dot = fcn(u,b,rr,rl)
%#codegen

wr = u(1);
wl = u(2);
theta = u(3);
sr = u(4);
sl = u(5);
x_dot = [((1-sl)*rl*wl + (1-sr)*rr*wr)*cos(theta)/2;
         ((1-sl)*rl*wl + (1-sr)*rr*wr)*sin(theta)/2;
         ((1-sl)*rl*wl - (1-sr)*rr*wr)/b];

== matlab function trackVehicleNewVer7_SonarPath/Tank/MATLAB Function1 ==
  data: obstacles input; rObst output; xUGV input; yUGV input; aUGV input; sonarInfo parameter
function rObst = sonarRange(obstacles,xUGV,yUGV,aUGV,sonarInfo)
%#codegen

% obstacles : Matrix 3Xn, n is the number of obstacles
% obstacles(1,:): x-position of obstacles [m]
% obstacles(2,:): y-position of obstacles [m]
% obstacles(3,:): radious of obstacles [m]

% xUGV:  x-position of UGV [m]
% yUGV:  y-position of UGV [m]
% aUGV: orientation of UGV [rad]


% sonarInfo.as : width of the sensor coveragle [m]
% sonarInfo.bs : length of the sensor coveragle [m]
% sonarInfo.hs : position of the sensor coveragle [m] (offset longitudinally from the origin of the body-frame)

% rObst: range of the obstacle measured by the sonar sensor [cm] !!!! note
% the unit.  unit is cm because that is what the actual sensor readings are

rObst = 7.67; % default sensor output when there is no detection

RBI = [cos(aUGV) sin(aUGV);-sin(aUGV) cos(aUGV)];


temp =size(obstacles);
noOfObst = temp(2);
for indexObst = 1:noOfObst
    
    rhoXYobst = RBI*(obstacles(1:2,indexObst)-[xUGV;yUGV]);
    
    obstXup    = rhoXYobst(1)+obstacles(3,indexObst);
    obstXdown  = rhoXYobst(1)-obstacles(3,indexObst);
    obstYright = rhoXYobst(2)+obstacles(3,indexObst);
    obstYleft  = rhoXYobst(2)-obstacles(3,indexObst);
    
    sonarXup    =  sonarInfo.hs + sonarInfo.bs;
    sonarXdown  =  sonarInfo.hs;
    sonarYright =  sonarInfo.as/2;
    sonarYleft  = -sonarInfo.as/2;
    
    flgOLx = overlapCheck([obstXdown obstXup],[sonarXdown sonarXup]);
    flgOLy = overlapCheck([obstYleft obstYright],[sonarYleft sonarYright]);
    
    if flgOLx && flgOLy
        temp2 = max(0,rhoXYobst(1) - obstacles(3,indexObst) - sonarInfo.hs);
        rObst = min(temp2,rObst);
    end
end
rObst = 100*rObst;


function [flgOL]=overlapCheck(aa,bb)
%#codegen
% checks if there is overlap between two intervals (aa(1),aa(2)) and (bb(1),bb(3))
% flgOL = 0 => no overlap, flgOL = 1 => overlap
% Dogan, 20150403

flgOL = 0;
if aa(1) <= bb(1)
    left = aa;
    right = bb;
else
    left = bb;
    right = aa;
end

if left(2) >= right(1)
    flgOL = 1;
end

== matlab function trackVehicleNewVer7_SonarPath/MATLAB Function1 ==
  data: tT input; sR output; sL output
function [sR,sL] = slipFnc(tT)
%#codegen

% tT  : time
% sR  : slippage on Right Track
% sL  : slippage on Left Track

% initialization
sR=0;sL=0;

% if tT > 10 && tT < 14
%     sL=0.4;
% end
%

== matlab function trackVehicleNewVer7_SonarPath/GNC/Guidance2/Path Planner/PathPlanner ==
  data: x input; y input; heading input; goals input; OccGrid input; path output; cellsize input; gridorig input; pathlen output
% Cartesian coordinate wrapper for path planner
% Start position: x, y
% Robot orientation: heading  - 0 is along the X-axis in a right-handed
% coordinate system
% goal: A list of alternative goal locations
% OccGrid: The occupancy grid - 0=Freedpace, 1=Obstacle, 2=Goal

function [path, pathlen] = PathPlanner(x, y, heading, goals, OccGrid, cellsize, gridorig)
path = zeros(size(OccGrid,1)*size(OccGrid,2),2);
pathlen = 0;
% Convert initial position to corresponding cell
ix = 0;
iy = 0;
[ix, iy] = pos2cell(x, y, cellsize, gridorig);

% Set goal states
if (size(goals, 1) > 0)
    for goalnum=1:size(goals, 1),
        [gx, gy] = pos2cell(goals(goalnum, 1), goals(goalnum, 2), cellsize, gridorig);
        OccGrid(gx, gy) = 3;
    end;
    
    % Plan the path on the discrete grid
    [cellpath, cellpathlen] = planPath(ix, iy, heading, OccGrid);

    % Set starting to beginning of the path
    path(pathlen+1,:) = [x, y]; 
    pathlen = pathlen+1; 
    if (cellpathlen > 0)   
        % Translate path into cartesian coordinates
        for step=1:cellpathlen,
            [tx, ty] = cell2pos(cellpath(step,1), cellpath(step,2), cellsize, gridorig);
            path(pathlen+1,:) = [tx, ty];
            pathlen = pathlen+1;
        end;
        % find nearest goal to goal bin and add it to the path as a final
        % location
        goalcell = [path(pathlen,1), path(pathlen,2)];
        mindist = Inf();
        goalindex = -1;
        for goalnum=1:size(goals, 1),
            tmpdist = sqrt((goalcell(1)-goals(goalnum,1))*(goalcell(1)-goals(goalnum,1)) + (goalcell(2)-goals(goalnum,2))*(goalcell(2)-goals(goalnum,2)));
            if (tmpdist < mindist)
                mindist = tmpdist;
                goalindex = goalnum;
            end;
        end;
        path(pathlen+1,:) = [goals(goalindex, 1), goals(goalindex, 2)];
        pathlen = pathlen + 1;
    end;
end;
path(1:pathlen,:)
end


% Path planner in grid cell coordinates
% Start grid cell: ix, iy
% Robot orientation: heading  - 0 is along the X-axis in a right-handed
% coordinate system
% OccGrid: The occupancy grid - 0=Freedpace, 1=Obstacle, 2=Goal
function [path, pathlen] = planPath(ix, iy, heading, OccGrid)
path = zeros(size(OccGrid, 1)*size(OccGrid, 2), 2);
pathlen = 0;
gridsize = size(OccGrid);

% This is the place for the actual path planner




end



% Converts cartesian position into grid cell index
function [ix, iy] = pos2cell(x, y, cellsize, gridorig)
ix = max(floor((x - gridorig(1))/cellsize(1))+1, 1);
iy = max(floor((y - gridorig(2))/cellsize(2))+1, 1);
end

%Converts grid cell index into cartesian position
function [x, y] = cell2pos(ix, iy, cellsize, gridorig)
x = (ix-0.5) * cellsize(1) + gridorig(1);
y = (iy-0.5) * cellsize(2) + gridorig(2);
end

== matlab function trackVehicleNewVer7_SonarPath/GNC/Guidance2/Waypoint Generator/Waypoint Sequencer ==
  data: x input; y input; path input; xway output; yway output; pathlen input; pathidx input; wayidx output; newpath input; stop output; maxwaydist input; maxgoaldist input
function [xway, yway, wayidx, stop] = NextWaypoint(x, y, path, pathlen, pathidx, newpath, maxwaydist, maxgoaldist)
xway = 0.0;
yway = 0.0;
wayidx = pathidx;
stop = 0;

if (pathlen > 0)
    if (newpath)
        wayidx = 1;
    end
    currdist = sqrt((path(wayidx, 1)-x)*(path(wayidx, 1)-x) + (path(wayidx, 2)-y)*(path(wayidx, 2)-y));
    if ( currdist < maxwaydist)
        if (wayidx == pathlen)
            if (currdist < maxgoaldist) 
                stop = 1;
            end
        else
            wayidx = wayidx + 1; 
        end
    end
    xway = path(wayidx, 1);
    yway = path(wayidx, 2);        
else
    xway = x;
    yway = y;
end;
end
